simulink library "matrix_visualizer"  (R2012b)
settings: Solver=ode45  StartTime=0.0  StopTime=10.0  RelTol=1e-3
settings Model: Creator=fede  LastModifiedBy=fede

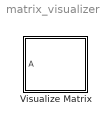
== system matrix_visualizer ==
  Visualize Matrix : MATLAB Function  TreatAsAtomicUnit=on

== matlab function matrix_visualizer/Visualize Matrix ==
  data: A input
function vis_matrix( A )
%#codegen
    
   coder.extrinsic('imagesc')
   coder.extrinsic('colorbar')
   
   persistent plot_h counter
   if isempty(counter)
       counter = 0;
   end   
   if isempty(plot_h)
       figure('doublebuffer','on')
       set(gca,'drawmode','fast');
       colormap('gray')   
       clims =  [-.05 0.3];
       plot_h = imagesc(zeros(25), clims);
       colorbar
   end
   
   if ~mod(counter, 15) 
       set(plot_h, 'CData', A);
   end
   counter = counter + 1;
end
